simulink model "v15_counters"  (R2019b)
settings: Solver=FixedStepAuto  StartTime=0.0  StopTime=100  FixedStep=1  MaxStep=1  RelTol=1e-3
libraries: simulink_extras x17
settings Model: Creator=MARAT  LastModifiedBy=Marat
settings SFSimCC: CustomCodeUndefinedFunction=UseInterfaceOnly

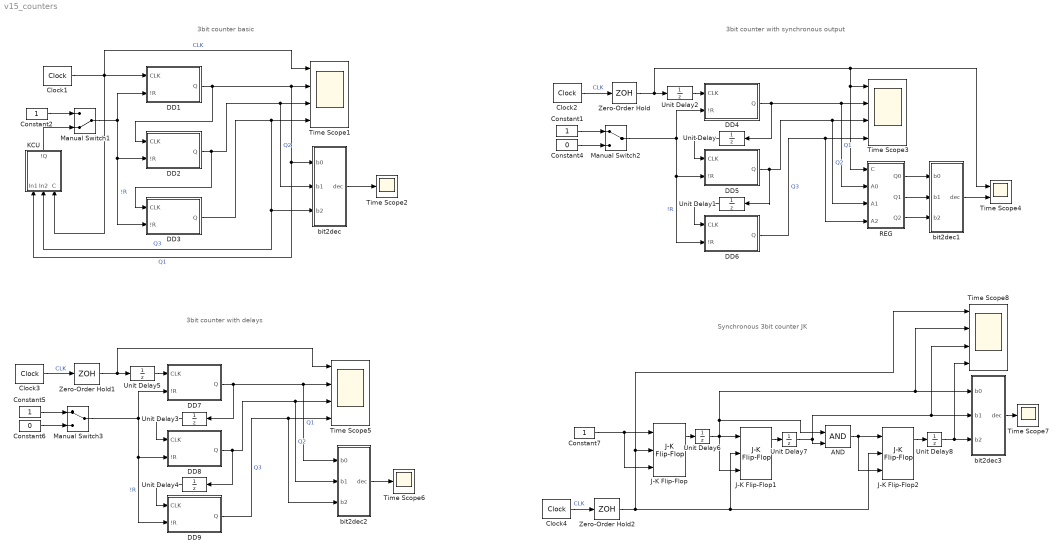
== system v15_counters ==
  note: 3bit counter with synchronous output
  note: 3bit counter basic
  note: 3bit counter with delays
  note: Synchronous 3bit counter JK
  AND : Logic  IconShape=distinctive  AllPortsSameDT=off  OutDataTypeStr=boolean
  Clock{1..4} (4 alike) : simulink_extras/Flip Flops/Clock  period=10
  Constant{1..2,5,7} (4 alike) : Constant  OutDataTypeStr=boolean
  Constant4 : Constant  Value=0  OutDataTypeStr=boolean
  Constant6 : Constant  Value=0  OutDataTypeStr=boolean
  DD1 : Subsystem
      mask Display: disp('TFF \nneg\nedge');
  DD2 : Subsystem
      mask Display: disp('TFF \nneg\nedge');
  DD3 : Subsystem
      mask Display: disp('TFF \nneg\nedge');
  DD4 : Subsystem
      mask Display: disp('TFF \nneg\nedge');
  DD5 : Subsystem
      mask Display: disp('TFF \nneg\nedge');
  DD6 : Subsystem
      mask Display: disp('TFF \nneg\nedge');
  DD7 : Subsystem
      mask Display: disp('TFF \nneg\nedge');
  DD8 : Subsystem
      mask Display: disp('TFF \nneg\nedge');
  DD9 : Subsystem
      mask Display: disp('TFF \nneg\nedge');
  J-K Flip-Flop : simulink_extras/Flip Flops/J-K Flip-Flop  initial_condition=0
      settings: SourceProductName=Simulink
  J-K Flip-Flop1 : simulink_extras/Flip Flops/J-K Flip-Flop  initial_condition=0
      settings: SourceProductName=Simulink
  J-K Flip-Flop2 : simulink_extras/Flip Flops/J-K Flip-Flop  initial_condition=0
      settings: SourceProductName=Simulink
  KCU : Subsystem
  Manual Switch1 : ManualSwitch  CurrentSetting=0
  Manual Switch2 : ManualSwitch
  Manual Switch3 : ManualSwitch
  REG : Subsystem
  Time Scope{1,3,5,8} (4 alike) : Scope  NumInputPorts=4
  Time Scope2 : Scope
  Time Scope4 : Scope  NumInputPorts=2
  Time Scope6 : Scope
  Time Scope7 : Scope
  Unit Delay{,1..8} (9 alike) : UnitDelay  SampleTime=-1  HasFrameUpgradeWarning=on
  Zero-Order Hold : ZeroOrderHold
  Zero-Order Hold1 : ZeroOrderHold
  Zero-Order Hold2 : ZeroOrderHold
  bit2dec : Subsystem
  bit2dec1 : Subsystem
  bit2dec2 : Subsystem
  bit2dec3 : Subsystem
  wires:
  Constant2/1 -> Manual Switch1/1
  Clock1/1 -> DD1/1(CLK), KCU/3(C), Time Scope1/1  "CLK"
  Manual Switch1/1 -> DD3/2(!R), DD2/2(!R), DD1/2(!R)  "!R"
  DD1/1(Q) -> DD2/1(CLK), KCU/1(In1), bit2dec/1(b0), Time Scope1/2  "Q1"
  DD2/1(Q) -> DD3/1(CLK), bit2dec/2(b1), Time Scope1/3  "Q2"
  DD3/1(Q) -> bit2dec/3(b2), KCU/2(In2), Time Scope1/4  "Q3"
  bit2dec/1(dec) -> Time Scope2/1
  DD6/1(Q) -> REG/4(A2), Time Scope3/4  "Q3"
  Manual Switch2/1 -> DD6/2(!R), DD5/2(!R), DD4/2(!R)  "!R"
  Constant4/1 -> Manual Switch2/2
  Constant1/1 -> Manual Switch2/1
  Clock2/1 -> Zero-Order Hold/1  "CLK"
  DD5/1(Q) -> Unit Delay1/1, REG/3(A1), Time Scope3/3  "Q2"
  DD4/1(Q) -> Unit Delay/1, REG/2(A0), Time Scope3/2  "Q1"
  Zero-Order Hold/1 -> Unit Delay2/1, Time Scope4/1, REG/1(C), Time Scope3/1
  Unit Delay/1 -> DD5/1(CLK)
  Unit Delay1/1 -> DD6/1(CLK)
  Unit Delay2/1 -> DD4/1(CLK)
  bit2dec1/1(dec) -> Time Scope4/2
  REG/1(Q0) -> bit2dec1/1(b0)
  REG/2(Q1) -> bit2dec1/2(b1)
  REG/3(Q2) -> bit2dec1/3(b2)
  bit2dec2/1(dec) -> Time Scope6/1
  Unit Delay5/1 -> DD7/1(CLK)
  Unit Delay4/1 -> DD9/1(CLK)
  Unit Delay3/1 -> DD8/1(CLK)
  Zero-Order Hold1/1 -> Time Scope5/1, Unit Delay5/1
  DD7/1(Q) -> bit2dec2/1(b0), Time Scope5/2, Unit Delay3/1  "Q1"
  DD8/1(Q) -> bit2dec2/2(b1), Time Scope5/3, Unit Delay4/1  "Q2"
  Clock3/1 -> Zero-Order Hold1/1  "CLK"
  Constant5/1 -> Manual Switch3/1
  Constant6/1 -> Manual Switch3/2
  Manual Switch3/1 -> DD7/2(!R), DD8/2(!R), DD9/2(!R)  "!R"
  DD9/1(Q) -> bit2dec2/3(b2), Time Scope5/4  "Q3"
  J-K Flip-Flop/1 -> Unit Delay6/1
  Constant7/1 -> J-K Flip-Flop/3, J-K Flip-Flop/1
  Clock4/1 -> Zero-Order Hold2/1  "CLK"
  J-K Flip-Flop2/1 -> Unit Delay8/1
  J-K Flip-Flop1/1 -> Unit Delay7/1
  AND/1 -> J-K Flip-Flop2/3, J-K Flip-Flop2/1
  bit2dec3/1(dec) -> Time Scope7/1
  Unit Delay6/1 -> AND/1, Time Scope8/2, bit2dec3/1(b0), J-K Flip-Flop1/3, J-K Flip-Flop1/1
  Unit Delay7/1 -> AND/2, Time Scope8/3, bit2dec3/2(b1)
  Unit Delay8/1 -> bit2dec3/3(b2), Time Scope8/4
  Zero-Order Hold2/1 -> J-K Flip-Flop1/2, J-K Flip-Flop2/2, J-K Flip-Flop/2, Time Scope8/1
  KCU/1(!Q) -> Manual Switch1/2

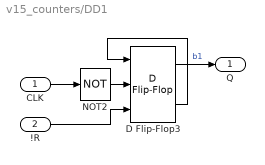
== system v15_counters/DD1 ==
  CLK : Inport
  !R : Inport  Port=2
  D Flip-Flop3 : simulink_extras/Flip Flops/D Flip-Flop
      settings: SourceProductName=Simulink
  NOT2 : Logic  Operator=NOT  IconShape=distinctive  AllPortsSameDT=off  OutDataTypeStr=boolean
  Q : Outport
  wires:
  D Flip-Flop3/2 -> D Flip-Flop3/1
  NOT2/1 -> D Flip-Flop3/2
  D Flip-Flop3/1 -> Q/1  "b1"
  CLK/1 -> NOT2/1
  !R/1 -> D Flip-Flop3/3

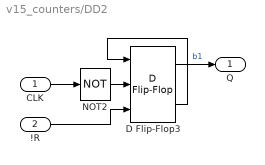
== system v15_counters/DD2 ==
  CLK : Inport
  !R : Inport  Port=2
  D Flip-Flop3 : simulink_extras/Flip Flops/D Flip-Flop
      settings: SourceProductName=Simulink
  NOT2 : Logic  Operator=NOT  IconShape=distinctive  AllPortsSameDT=off  OutDataTypeStr=boolean
  Q : Outport
  wires:
  !R/1 -> D Flip-Flop3/3
  CLK/1 -> NOT2/1
  D Flip-Flop3/1 -> Q/1  "b1"
  NOT2/1 -> D Flip-Flop3/2
  D Flip-Flop3/2 -> D Flip-Flop3/1

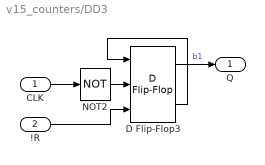
== system v15_counters/DD3 ==
  CLK : Inport
  !R : Inport  Port=2
  D Flip-Flop3 : simulink_extras/Flip Flops/D Flip-Flop
      settings: SourceProductName=Simulink
  NOT2 : Logic  Operator=NOT  IconShape=distinctive  AllPortsSameDT=off  OutDataTypeStr=boolean
  Q : Outport
  wires:
  D Flip-Flop3/2 -> D Flip-Flop3/1
  NOT2/1 -> D Flip-Flop3/2
  D Flip-Flop3/1 -> Q/1  "b1"
  CLK/1 -> NOT2/1
  !R/1 -> D Flip-Flop3/3

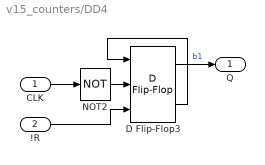
== system v15_counters/DD4 ==
  CLK : Inport
  !R : Inport  Port=2
  D Flip-Flop3 : simulink_extras/Flip Flops/D Flip-Flop
      settings: SourceProductName=Simulink
  NOT2 : Logic  Operator=NOT  IconShape=distinctive  AllPortsSameDT=off  OutDataTypeStr=boolean
  Q : Outport
  wires:
  D Flip-Flop3/2 -> D Flip-Flop3/1
  NOT2/1 -> D Flip-Flop3/2
  D Flip-Flop3/1 -> Q/1  "b1"
  CLK/1 -> NOT2/1
  !R/1 -> D Flip-Flop3/3

== system v15_counters/DD5 ==
  CLK : Inport
  !R : Inport  Port=2
  D Flip-Flop3 : simulink_extras/Flip Flops/D Flip-Flop
      settings: SourceProductName=Simulink
  NOT2 : Logic  Operator=NOT  IconShape=distinctive  AllPortsSameDT=off  OutDataTypeStr=boolean
  Q : Outport
  wires:
  !R/1 -> D Flip-Flop3/3
  CLK/1 -> NOT2/1
  D Flip-Flop3/1 -> Q/1  "b1"
  NOT2/1 -> D Flip-Flop3/2
  D Flip-Flop3/2 -> D Flip-Flop3/1

== system v15_counters/DD6 ==
  CLK : Inport
  !R : Inport  Port=2
  D Flip-Flop3 : simulink_extras/Flip Flops/D Flip-Flop
      settings: SourceProductName=Simulink
  NOT2 : Logic  Operator=NOT  IconShape=distinctive  AllPortsSameDT=off  OutDataTypeStr=boolean
  Q : Outport
  wires:
  D Flip-Flop3/2 -> D Flip-Flop3/1
  NOT2/1 -> D Flip-Flop3/2
  D Flip-Flop3/1 -> Q/1  "b1"
  CLK/1 -> NOT2/1
  !R/1 -> D Flip-Flop3/3

== system v15_counters/DD7 ==
  CLK : Inport
  !R : Inport  Port=2
  D Flip-Flop3 : simulink_extras/Flip Flops/D Flip-Flop
      settings: SourceProductName=Simulink
  NOT2 : Logic  Operator=NOT  IconShape=distinctive  AllPortsSameDT=off  OutDataTypeStr=boolean
  Q : Outport
  wires:
  !R/1 -> D Flip-Flop3/3
  CLK/1 -> NOT2/1
  D Flip-Flop3/1 -> Q/1  "b1"
  NOT2/1 -> D Flip-Flop3/2
  D Flip-Flop3/2 -> D Flip-Flop3/1

== system v15_counters/DD8 ==
  CLK : Inport
  !R : Inport  Port=2
  D Flip-Flop3 : simulink_extras/Flip Flops/D Flip-Flop
      settings: SourceProductName=Simulink
  NOT2 : Logic  Operator=NOT  IconShape=distinctive  AllPortsSameDT=off  OutDataTypeStr=boolean
  Q : Outport
  wires:
  D Flip-Flop3/2 -> D Flip-Flop3/1
  NOT2/1 -> D Flip-Flop3/2
  D Flip-Flop3/1 -> Q/1  "b1"
  CLK/1 -> NOT2/1
  !R/1 -> D Flip-Flop3/3

== system v15_counters/DD9 ==
  CLK : Inport
  !R : Inport  Port=2
  D Flip-Flop3 : simulink_extras/Flip Flops/D Flip-Flop
      settings: SourceProductName=Simulink
  NOT2 : Logic  Operator=NOT  IconShape=distinctive  AllPortsSameDT=off  OutDataTypeStr=boolean
  Q : Outport
  wires:
  !R/1 -> D Flip-Flop3/3
  CLK/1 -> NOT2/1
  D Flip-Flop3/1 -> Q/1  "b1"
  NOT2/1 -> D Flip-Flop3/2
  D Flip-Flop3/2 -> D Flip-Flop3/1

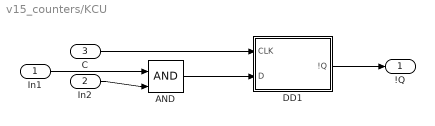
== system v15_counters/KCU ==
  In1 : Inport
  In2 : Inport  Port=2
  C : Inport  Port=3
  AND : Logic  IconShape=distinctive  AllPortsSameDT=off  OutDataTypeStr=boolean
  DD1 : Subsystem
      mask Display: disp('DFF \nneg\nedge');
  !Q : Outport
  wires:
  DD1/1(!Q) -> !Q/1
  In1/1 -> AND/1
  In2/1 -> AND/2
  AND/1 -> DD1/2(D)
  C/1 -> DD1/1(CLK)

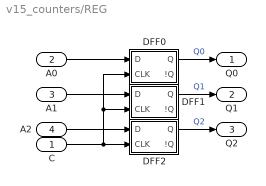
== system v15_counters/REG ==
  C : Inport
  A0 : Inport  Port=2
  A1 : Inport  Port=3
  A2 : Inport  Port=4
  DFF0 : Subsystem
  DFF1 : Subsystem
  DFF2 : Subsystem
  Q0 : Outport
  Q1 : Outport  Port=2
  Q2 : Outport  Port=3
  wires:
  DFF1/1(Q) -> Q1/1  "Q1"
  A2/1 -> DFF2/1(D)
  C/1 -> DFF2/2(CLK), DFF1/2(CLK), DFF0/2(CLK)
  A1/1 -> DFF1/1(D)
  DFF0/1(Q) -> Q0/1  "Q0"
  A0/1 -> DFF0/1(D)
  DFF2/1(Q) -> Q2/1  "Q2"

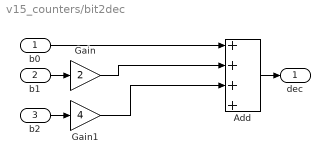
== system v15_counters/bit2dec ==
  b0 : Inport
  b1 : Inport  Port=2
  b2 : Inport  Port=3
  Add : Sum  Inputs=++++
  Gain : Gain  Gain=2
  Gain1 : Gain  Gain=4
  dec : Outport
  wires:
  b1/1 -> Gain/1
  b2/1 -> Gain1/1
  b0/1 -> Add/1
  Add/1 -> dec/1
  Gain/1 -> Add/2
  Gain1/1 -> Add/3

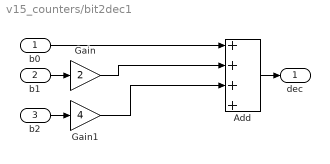
== system v15_counters/bit2dec1 ==
  b0 : Inport
  b1 : Inport  Port=2
  b2 : Inport  Port=3
  Add : Sum  Inputs=++++
  Gain : Gain  Gain=2
  Gain1 : Gain  Gain=4
  dec : Outport
  wires:
  Gain1/1 -> Add/3
  Gain/1 -> Add/2
  Add/1 -> dec/1
  b0/1 -> Add/1
  b2/1 -> Gain1/1
  b1/1 -> Gain/1

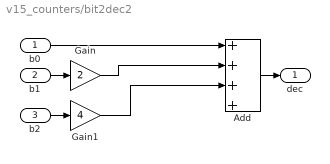
== system v15_counters/bit2dec2 ==
  b0 : Inport
  b1 : Inport  Port=2
  b2 : Inport  Port=3
  Add : Sum  Inputs=++++
  Gain : Gain  Gain=2
  Gain1 : Gain  Gain=4
  dec : Outport
  wires:
  b1/1 -> Gain/1
  b2/1 -> Gain1/1
  b0/1 -> Add/1
  Add/1 -> dec/1
  Gain/1 -> Add/2
  Gain1/1 -> Add/3

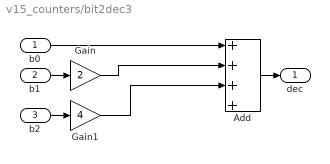
== system v15_counters/bit2dec3 ==
  b0 : Inport
  b1 : Inport  Port=2
  b2 : Inport  Port=3
  Add : Sum  Inputs=++++
  Gain : Gain  Gain=2
  Gain1 : Gain  Gain=4
  dec : Outport
  wires:
  Gain1/1 -> Add/3
  Gain/1 -> Add/2
  Add/1 -> dec/1
  b0/1 -> Add/1
  b2/1 -> Gain1/1
  b1/1 -> Gain/1

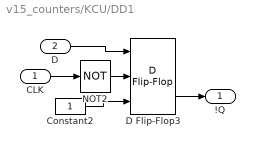
== system v15_counters/KCU/DD1 ==
  CLK : Inport
  D : Inport  Port=2
  Constant2 : Constant  OutDataTypeStr=boolean
  D Flip-Flop3 : simulink_extras/Flip Flops/D Flip-Flop
      settings: SourceProductName=Simulink
  NOT2 : Logic  Operator=NOT  IconShape=distinctive  AllPortsSameDT=off  OutDataTypeStr=boolean
  !Q : Outport
  wires:
  NOT2/1 -> D Flip-Flop3/2
  CLK/1 -> NOT2/1
  Constant2/1 -> D Flip-Flop3/3
  D/1 -> D Flip-Flop3/1
  D Flip-Flop3/2 -> !Q/1

== system v15_counters/REG/DFF0 ==
  D : Inport
  CLK : Inport  Port=2
  Subsystem : Subsystem
  Q : Outport  InitialOutput=0  VectorParamsAs1DForOutWhenUnconnected=off
  !Q : Outport  Port=2  InitialOutput=1  VectorParamsAs1DForOutWhenUnconnected=off
  wires:
  Subsystem/2(!Q) -> !Q/1
  Subsystem/1(Q) -> Q/1
  D/1 -> Subsystem/1(D)
  CLK/1 -> Subsystem/Trigger

== system v15_counters/REG/DFF1 ==
  D : Inport
  CLK : Inport  Port=2
  Subsystem : Subsystem
  Q : Outport  InitialOutput=0  VectorParamsAs1DForOutWhenUnconnected=off
  !Q : Outport  Port=2  InitialOutput=1  VectorParamsAs1DForOutWhenUnconnected=off
  wires:
  CLK/1 -> Subsystem/Trigger
  D/1 -> Subsystem/1(D)
  Subsystem/1(Q) -> Q/1
  Subsystem/2(!Q) -> !Q/1

== system v15_counters/REG/DFF2 ==
  D : Inport
  CLK : Inport  Port=2
  Subsystem : Subsystem
  Q : Outport  InitialOutput=0  VectorParamsAs1DForOutWhenUnconnected=off
  !Q : Outport  Port=2  InitialOutput=1  VectorParamsAs1DForOutWhenUnconnected=off
  wires:
  Subsystem/2(!Q) -> !Q/1
  Subsystem/1(Q) -> Q/1
  D/1 -> Subsystem/1(D)
  CLK/1 -> Subsystem/Trigger

== system v15_counters/REG/DFF0/Subsystem ==
  D : Inport  LatchByDelayingOutsideSignal=on
  Trigger : TriggerPort  VariantControl=Variant  StatesWhenEnabling=reset
  Logic : Logic  Operator=NOT  Inputs=1
  Q : Outport  OutputWhenDisabled=reset  InitialOutput=0  VectorParamsAs1DForOutWhenUnconnected=off
  !Q : Outport  Port=2  OutputWhenDisabled=reset  InitialOutput=1  VectorParamsAs1DForOutWhenUnconnected=off
  wires:
  D/1 -> Logic/1, Q/1
  Logic/1 -> !Q/1

== system v15_counters/REG/DFF1/Subsystem ==
  D : Inport  LatchByDelayingOutsideSignal=on
  Trigger : TriggerPort  VariantControl=Variant  StatesWhenEnabling=reset
  Logic : Logic  Operator=NOT  Inputs=1
  Q : Outport  OutputWhenDisabled=reset  InitialOutput=0  VectorParamsAs1DForOutWhenUnconnected=off
  !Q : Outport  Port=2  OutputWhenDisabled=reset  InitialOutput=1  VectorParamsAs1DForOutWhenUnconnected=off
  wires:
  Logic/1 -> !Q/1
  D/1 -> Q/1, Logic/1

== system v15_counters/REG/DFF2/Subsystem ==
  D : Inport  LatchByDelayingOutsideSignal=on
  Trigger : TriggerPort  VariantControl=Variant  StatesWhenEnabling=reset
  Logic : Logic  Operator=NOT  Inputs=1
  Q : Outport  OutputWhenDisabled=reset  InitialOutput=0  VectorParamsAs1DForOutWhenUnconnected=off
  !Q : Outport  Port=2  OutputWhenDisabled=reset  InitialOutput=1  VectorParamsAs1DForOutWhenUnconnected=off
  wires:
  D/1 -> Logic/1, Q/1
  Logic/1 -> !Q/1
